simulink library "TYPEBP_MASTER_tmp"  (Simulink 8.6)
settings: Solver=ode45  StartTime=0.0  StopTime=10.0  RelTol=1e-3
undefined symbols (not defined in the file): TYPEC, TYPEC_MASTER
libraries: cdsEpicsOut x112, cdsFilt x79, cdsTP x59, cdsFiltCtrl x36, VIS_LIB x20, cdsEpicsIn x18, cdsMuxMatrix x14, STATE_BIO_MASTER x12, cdsEpicsBinIn x8, cdsFunctionCall x4, lockin x4, cdsEpicsStringIn x2
(part 2 of 13)

== system TYPEBP_MASTER_tmp/TYPEBPMASTER/TEST ==
  In1 : Inport
  In4 : Inport  Port=2
  In7 : Inport  Port=3
  In10 : Inport  Port=4
  CH1 : cdsFiltCtrl/IIR FM with control  Tag=cdsFiltCtrl  Description=|
      | cdsFiltCntrl is the standard IIR filter module (exactly the same as cdsFilt) but with added control data output 'Ctrl'. Filter module digital signal output appears on the first output, which is called 'Val'. 'Ctrl' output has a bit pattern encoding the state of filter's on/off switches (FM1 through FM10). The bit values are:
      |                                                                                                                                                                                                                                                                                                                                       
      | module 	hex	dec                                                                                                                                                                                                                                                                                                                       
      | -----------------------                                                                                                                                                                                                                                                                                                               
      | FM1	0x20                    32                                                                                                                                                                                                                                                                                                        
      | FM2	0x80                     128                                                                                                                                                                                                                                                                                                      
      | FM3	0x200                   512                                                                                                                                                                                                                                                                                                       
      | FM4	0x800                   2048                                                                                                                                                                                                                                                                                                      
      | FM5	0x2000                 8192                                                                                                                                                                                                                                                                                                       
      | FM6	0x8000                 32768                                                                                                                                                                                                                                                                                                      
      | FM7	0x20000                131072                                                                                                                                                                                                                                                                                                     
      | FM8	0x80000                 524288                                                                                                                                                                                                                                                                                                    
      | FM9	0x200000               2097152                                                                                                                                                                                                                                                                                                    
      | FM10	0x800000               8388608                                                                                                                                                                                                                                                                                                   
      |                                                                                                                                                                                                                                                                                                                                       
      | This bit data can be used to drive some other switches or it can be output using a binary I/O module.
      settings: AttributesFormatString=%<Tag>
  CH2 : cdsFiltCtrl/IIR FM with control  Tag=cdsFiltCtrl  Description=|
      | cdsFiltCntrl is the standard IIR filter module (exactly the same as cdsFilt) but with added control data output 'Ctrl'. Filter module digital signal output appears on the first output, which is called 'Val'. 'Ctrl' output has a bit pattern encoding the state of filter's on/off switches (FM1 through FM10). The bit values are:
      |                                                                                                                                                                                                                                                                                                                                       
      | module 	hex	dec                                                                                                                                                                                                                                                                                                                       
      | -----------------------                                                                                                                                                                                                                                                                                                               
      | FM1	0x20                    32                                                                                                                                                                                                                                                                                                        
      | FM2	0x80                     128                                                                                                                                                                                                                                                                                                      
      | FM3	0x200                   512                                                                                                                                                                                                                                                                                                       
      | FM4	0x800                   2048                                                                                                                                                                                                                                                                                                      
      | FM5	0x2000                 8192                                                                                                                                                                                                                                                                                                       
      | FM6	0x8000                 32768                                                                                                                                                                                                                                                                                                      
      | FM7	0x20000                131072                                                                                                                                                                                                                                                                                                     
      | FM8	0x80000                 524288                                                                                                                                                                                                                                                                                                    
      | FM9	0x200000               2097152                                                                                                                                                                                                                                                                                                    
      | FM10	0x800000               8388608                                                                                                                                                                                                                                                                                                   
      |                                                                                                                                                                                                                                                                                                                                       
      | This bit data can be used to drive some other switches or it can be output using a binary I/O module.
      settings: AttributesFormatString=%<Tag>
  CH3 : cdsFiltCtrl/IIR FM with control  Tag=cdsFiltCtrl  Description=|
      | cdsFiltCntrl is the standard IIR filter module (exactly the same as cdsFilt) but with added control data output 'Ctrl'. Filter module digital signal output appears on the first output, which is called 'Val'. 'Ctrl' output has a bit pattern encoding the state of filter's on/off switches (FM1 through FM10). The bit values are:
      |                                                                                                                                                                                                                                                                                                                                       
      | module 	hex	dec                                                                                                                                                                                                                                                                                                                       
      | -----------------------                                                                                                                                                                                                                                                                                                               
      | FM1	0x20                    32                                                                                                                                                                                                                                                                                                        
      | FM2	0x80                     128                                                                                                                                                                                                                                                                                                      
      | FM3	0x200                   512                                                                                                                                                                                                                                                                                                       
      | FM4	0x800                   2048                                                                                                                                                                                                                                                                                                      
      | FM5	0x2000                 8192                                                                                                                                                                                                                                                                                                       
      | FM6	0x8000                 32768                                                                                                                                                                                                                                                                                                      
      | FM7	0x20000                131072                                                                                                                                                                                                                                                                                                     
      | FM8	0x80000                 524288                                                                                                                                                                                                                                                                                                    
      | FM9	0x200000               2097152                                                                                                                                                                                                                                                                                                    
      | FM10	0x800000               8388608                                                                                                                                                                                                                                                                                                   
      |                                                                                                                                                                                                                                                                                                                                       
      | This bit data can be used to drive some other switches or it can be output using a binary I/O module.
      settings: AttributesFormatString=%<Tag>
  CH4 : cdsFiltCtrl/IIR FM with control  Tag=cdsFiltCtrl  Description=|
      | cdsFiltCntrl is the standard IIR filter module (exactly the same as cdsFilt) but with added control data output 'Ctrl'. Filter module digital signal output appears on the first output, which is called 'Val'. 'Ctrl' output has a bit pattern encoding the state of filter's on/off switches (FM1 through FM10). The bit values are:
      |                                                                                                                                                                                                                                                                                                                                       
      | module 	hex	dec                                                                                                                                                                                                                                                                                                                       
      | -----------------------                                                                                                                                                                                                                                                                                                               
      | FM1	0x20                    32                                                                                                                                                                                                                                                                                                        
      | FM2	0x80                     128                                                                                                                                                                                                                                                                                                      
      | FM3	0x200                   512                                                                                                                                                                                                                                                                                                       
      | FM4	0x800                   2048                                                                                                                                                                                                                                                                                                      
      | FM5	0x2000                 8192                                                                                                                                                                                                                                                                                                       
      | FM6	0x8000                 32768                                                                                                                                                                                                                                                                                                      
      | FM7	0x20000                131072                                                                                                                                                                                                                                                                                                     
      | FM8	0x80000                 524288                                                                                                                                                                                                                                                                                                    
      | FM9	0x200000               2097152                                                                                                                                                                                                                                                                                                    
      | FM10	0x800000               8388608                                                                                                                                                                                                                                                                                                   
      |                                                                                                                                                                                                                                                                                                                                       
      | This bit data can be used to drive some other switches or it can be output using a binary I/O module.
      settings: AttributesFormatString=%<Tag>
  Ground{1..6,19,22} (8 alike) : Ground
  Terminator{1..5,16..18} (8 alike) : Terminator
  wires:
  CH1/1 -> Terminator5/1
  CH3/1 -> Terminator3/1
  CH4/1 -> Terminator2/1
  In4/1 -> CH2/1
  CH2/1 -> Terminator4/1
  In1/1 -> CH1/1
  In7/1 -> CH3/1
  In10/1 -> CH4/1
  Ground22/1 -> CH1/2
  Ground19/1 -> CH1/3
  CH1/2 -> Terminator16/1
  CH2/2 -> Terminator17/1
  CH3/2 -> Terminator18/1
  Ground2/1 -> CH2/2
  Ground1/1 -> CH2/3
  Ground4/1 -> CH3/2
  Ground3/1 -> CH3/3
  Ground6/1 -> CH4/2
  Ground5/1 -> CH4/3
  CH4/2 -> Terminator1/1

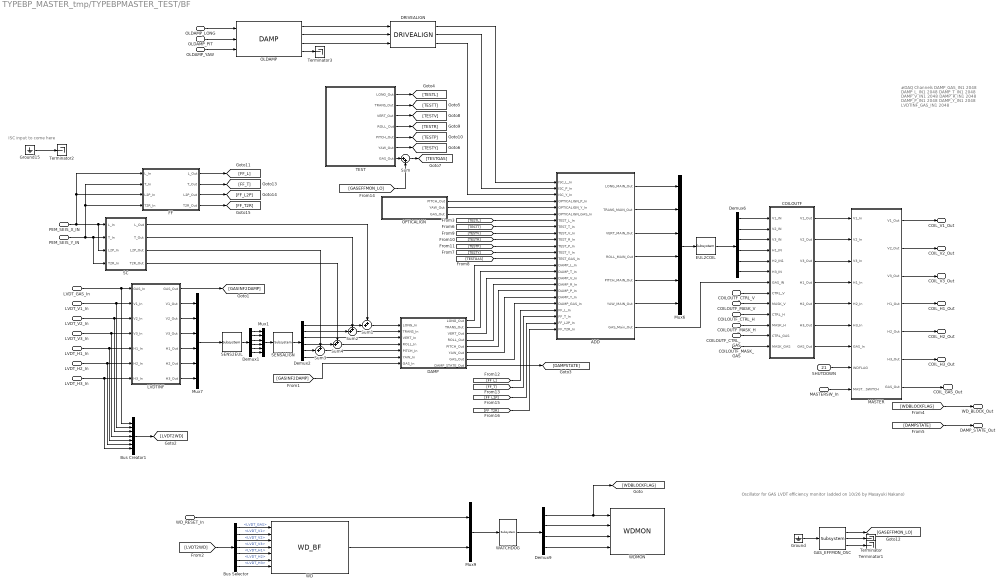
== system TYPEBP_MASTER_tmp/TYPEBPMASTER_TEST/BF ==
  note: #DAQ Channels
      | DAMP_GAS_IN1 2048
      | DAMP_L_IN1 2048
      | DAMP_T_IN1 2048
      | DAMP_V_IN1 2048
      | DAMP_R_IN1 2048
      | DAMP_P_IN1 2048
      | DAMP_Y_IN1 2048
      | LVDTINF_GAS_IN1 2048
  note: ISC input to come here
  note: Oscillator for GAS LVDT efficiency monitor (added on 10/26 by Masayuki Nakano)
  LVDT_GAS_In : Inport
  LVDT_V1_In : Inport  Port=2
  LVDT_V2_In : Inport  Port=3
  LVDT_V3_In : Inport  Port=4
  LVDT_H1_In : Inport  Port=5
  LVDT_H2_In : Inport  Port=6
  LVDT_H3_In : Inport  Port=7
  COILOUTF_CTRL_V : Inport  Port=8
  COILOUTF_MASK_V : Inport  Port=9
  COILOUTF_CTRL_H : Inport  Port=10
  COILOUTF_MASK_H : Inport  Port=11
  COILOUTF_CTRL_GAS : Inport  Port=12
  COILOUTF_MASK_GAS : Inport  Port=13
  MASTERSW_In : Inport  Port=14
  WD_RESET_In : Inport  Port=15
  OLDAMP_LONG : Inport  Port=16
  OLDAMP_PIT : Inport  Port=17
  OLDAMP_YAW : Inport  Port=18
  PEM_SEIS_X_IN : Inport  Port=19
  PEM_SEIS_Y_IN : Inport  Port=20
  SHUTDOWN : Inport  Port=21
  ADD : Subsystem
  Bus Creator1 : BusCreator  Inputs='LVDT_GAS','LVDT_V1','LVDT_V2','LVDT_V3','LVDT_H1','LVDT_H2','LVDT_H3'
  Bus Selector : BusSelector  OutputSignals=LVDT_GAS,LVDT_V1,LVDT_V2,LVDT_V3,LVDT_H1,LVDT_H2,LVDT_H3
  COILOUTF : Subsystem
  DAMP : Subsystem
  DRIVEALIGN : CRYP_IM_MASTER/CRYP_IM_MASTER/DRIVEALIGN
  Demux1 : Demux  Outputs=6
  Demux2 : Demux  Outputs=6
  Demux6 : Demux  Outputs=6
  Demux9 : Demux
  EUL2COIL : cdsMuxMatrix/Subsystem  Tag=cdsMuxMatrix  Description=|
      | ADL=SUS_INMATRIX.adl
      | SCRIPT=generate_KisselButton.py 4 5 #CHANNEL# > #TARGET_DIR#/#FULL_PART_NAME#_KB.adl
      settings: AttributesFormatString=%<Tag>
  FF : Subsystem  AncestorBlock=TYPEBP_MASTER/TYPEBPMASTER_TEST/SF/FF
  GAS_EFFMON_OSC : cdsOsc/Subsystem  Tag=cdsOsc  Description=Oscillator
      settings: AttributesFormatString=%<Tag>
  Ground : Ground
  Ground15 : Ground
  LVDTINF : Subsystem
  MASTER : Subsystem
  Mux1 : Mux  Inputs=6
  Mux6 : Mux  Inputs=6
  Mux7 : Mux  Inputs=6
  Mux9 : Mux  Inputs=2
  OLDAMP : VIS_LIB/DAMP
  OPTICALIGN : Subsystem
  SC : Subsystem
  SENS2EUL : cdsMuxMatrix/Subsystem  Tag=cdsMuxMatrix  Description=Any size matrix. Inputs and outputs must be connected using Mux and Demux parts.
      settings: AttributesFormatString=%<Tag>
  SENSALIGN : cdsMuxMatrix/Subsystem  Tag=cdsMuxMatrix  Description=Any size matrix. Inputs and outputs must be connected using Mux and Demux parts.
      settings: AttributesFormatString=%<Tag>
  Sum : Sum  Inputs=|++
  Sum{1..4} (4 alike) : Sum  Inputs=++|
  TEST : Subsystem
  Terminator{,1..3} (4 alike) : Terminator
  WATCHDOG : cdsFunctionCall/Subsystem  Tag=cdsFunctionCall  Description=inline OSEMWATCHDOG /opt/rtcds/userapps/release/vis/common/src/WATCHDOG.c
      settings: AttributesFormatString=%<Tag>\n%<Description>
  WD : VIS_LIB/WD_BF
  WDMON : SIXOSEM_F_STAGE_MASTER/SIXOSEM_F_STAGE_MASTER/WDMON
  COIL_GAS_Out : Outport
  COIL_V1_Out : Outport  Port=2
  COIL_V2_Out : Outport  Port=3
  COIL_V3_Out : Outport  Port=4
  COIL_H1_Out : Outport  Port=5
  COIL_H2_Out : Outport  Port=6
  COIL_H3_Out : Outport  Port=7
  WD_BLOCK_Out : Outport  Port=8
  DAMP_STATE_Out : Outport  Port=9
  wires:
  SC/4(T2R_Out) -> Sum4/1
  Sum4/1 -> DAMP/4(ROLL_In)
  SC/3(L2P_Out) -> Sum3/1
  Sum3/1 -> DAMP/5(PITCH_In)
  [FF_T2R] -> ADD/24(FF_T2R_In)
  [FF_L2P] -> ADD/23(FF_L2P_In)
  FF/4(T2R_Out) -> [FF_T2R]
  FF/3(L2P_Out) -> [FF_L2P]
  [FF_T] -> ADD/22(FF_T_In)
  [FF_L] -> ADD/21(FF_L_In)
  FF/2(T_Out) -> [FF_T]
  FF/1(L_Out) -> [FF_L]
  PEM_SEIS_X_IN/1 -> SC/1(L_In), SC/3(L2P_In), FF/3(L2P_In), FF/1(L_In)
  Sum2/1 -> DAMP/2(TRANS_In)
  Sum1/1 -> DAMP/1(LONG_In)
  SC/2(T_Out) -> Sum2/1
  PEM_SEIS_Y_IN/1 -> FF/2(T_In), FF/4(T2R_In), SC/2(T_In), SC/4(T2R_In)
  SC/1(L_Out) -> Sum1/1
  DRIVEALIGN/1 -> ADD/1(ISC_L_In)
  DRIVEALIGN/2 -> ADD/2(ISC_P_In)
  DRIVEALIGN/3 -> ADD/3(ISC_Y_In)
  OLDAMP/3 -> DRIVEALIGN/3
  OLDAMP/2 -> DRIVEALIGN/2
  OLDAMP/1 -> DRIVEALIGN/1
  Ground15/1 -> Terminator2/1
  OLDAMP_LONG/1 -> OLDAMP/1
  OLDAMP_PIT/1 -> OLDAMP/2
  OLDAMP_YAW/1 -> OLDAMP/3
  OLDAMP/4 -> Terminator3/1
  GAS_EFFMON_OSC/3 -> Terminator1/1
  GAS_EFFMON_OSC/2 -> Terminator/1
  Ground/1 -> GAS_EFFMON_OSC/1
  [GASEFFMON_LO] -> Sum/2
  Sum/1 -> [TESTGAS]
  TEST/7(GAS_Out) -> Sum/1
  GAS_EFFMON_OSC/1 -> [GASEFFMON_LO]
  [GASINF2DAMP] -> DAMP/7(GAS_In)
  COILOUTF_MASK_GAS/1 -> COILOUTF/13(MASK_GAS)
  COILOUTF_CTRL_GAS/1 -> COILOUTF/12(CTRL_GAS)
  COILOUTF_MASK_H/1 -> COILOUTF/11(MASK_H)
  COILOUTF_CTRL_H/1 -> COILOUTF/10(CTRL_H)
  LVDTINF/7(H3_Out) -> Mux7/6
  LVDTINF/6(H2_Out) -> Mux7/5
  LVDTINF/5(H1_Out) -> Mux7/4
  Bus Selector/7 -> WD/7  "<LVDT_H3>"
  Bus Selector/6 -> WD/6  "<LVDT_H2>"
  Bus Selector/5 -> WD/5  "<LVDT_H1>"
  Bus Selector/4 -> WD/4  "<LVDT_V3>"
  Bus Selector/3 -> WD/3  "<LVDT_V2>"
  Bus Selector/2 -> WD/2  "<LVDT_V1>"
  [DAMPSTATE] -> DAMP_STATE_Out/1
  [WDBLOCKFLAG] -> WD_BLOCK_Out/1
  MASTER/7(GAS_Out) -> COIL_GAS_Out/1
  MASTER/6(H3_Out) -> COIL_H3_Out/1
  MASTER/5(H2_Out) -> COIL_H2_Out/1
  MASTERSW_In/1 -> MASTER/9(MASTERSWITCH)
  SHUTDOWN/1 -> MASTER/8(WDFLAG)
  COILOUTF/4(H1_Out) -> MASTER/4(H1_In)
  COILOUTF/3(V3_Out) -> MASTER/3(V3_In)
  COILOUTF/2(V2_Out) -> MASTER/2(V2_In)
  COILOUTF/1(V1_Out) -> MASTER/1(V1_In)
  COILOUTF/7(GAS_Out) -> MASTER/7(GAS_In)
  COILOUTF/6(H3_Out) -> MASTER/6(H3_In)
  COILOUTF/5(H2_Out) -> MASTER/5(H2_In)
  Demux6/6 -> COILOUTF/6(H3_IN)
  Demux6/5 -> COILOUTF/5(H2_IN1)
  Demux6/4 -> COILOUTF/4(H1_IN)
  Demux6/3 -> COILOUTF/3(V3_IN)
  Demux6/2 -> COILOUTF/2(V2_IN)
  Demux6/1 -> COILOUTF/1(V1_IN)
  OPTICALIGN/3(GAS_Out) -> ADD/6(OPTICALIGN_GAS_In)
  OPTICALIGN/2(YAW_Out) -> ADD/5(OPTICALIGN_Y_In)
  OPTICALIGN/1(PITCH_Out) -> ADD/4(OPTICALIGN_P_In)
  ADD/1(LONG_MAIN_Out) -> Mux6/1
  ADD/2(TRANS_MAIN_Out) -> Mux6/2
  ADD/3(VERT_MAIN_Out) -> Mux6/3
  ADD/4(ROLL_MAIN_Out) -> Mux6/4
  ADD/5(PITCH_MAIN_Out) -> Mux6/5
  ADD/6(YAW_MAIN_Out) -> Mux6/6
  ADD/7(GAS_Main_Out) -> COILOUTF/7(GAS_IN)
  DAMP/1(LONG_Out) -> ADD/14(DAMP_L_In)
  DAMP/2(TRANS_Out) -> ADD/15(DAMP_T_In)
  DAMP/3(VERT_Out) -> ADD/16(DAMP_V_In)
  DAMP/4(ROLL_Out) -> ADD/17(DAMP_R_In)
  DAMP/5(PITCH_Out) -> ADD/18(DAMP_P_In)
  DAMP/6(YAW_Out) -> ADD/19(DAMP_Y_In)
  DAMP/7(GAS_Out) -> ADD/20(DAMP_GAS_In)
  [TESTP] -> ADD/11(TEST_P_In)
  [TESTR] -> ADD/10(TEST_R_In)
  [TESTV] -> ADD/9(TEST_V_In)
  TEST/5(PITCH_Out) -> [TESTP]
  TEST/4(ROLL_Out) -> [TESTR]
  TEST/3(VERT_Out) -> [TESTV]
  DAMP/8(DAMP_STATE_Out) -> [DAMPSTATE]
  LVDTINF/4(V3_Out) -> Mux7/3
  LVDTINF/3(V2_Out) -> Mux7/2
  LVDTINF/2(V1_Out) -> Mux7/1
  SENSALIGN/1 -> Demux2/1
  Mux1/1 -> SENSALIGN/1
  Demux1/6 -> Mux1/6
  Demux1/5 -> Mux1/5
  Demux1/4 -> Mux1/4
  Demux1/3 -> Mux1/3
  Demux1/2 -> Mux1/2
  Demux1/1 -> Mux1/1
  SENS2EUL/1 -> Demux1/1
  Demux2/1 -> Sum1/2
  Demux2/2 -> Sum2/2
  Demux2/3 -> DAMP/3(VERT_In)
  Demux2/4 -> Sum4/2
  Demux2/5 -> Sum3/2
  Demux2/6 -> DAMP/6(YAW_In)
  Bus Selector/1 -> WD/1  "<LVDT_GAS>"
  MASTER/4(H1_Out) -> COIL_H1_Out/1
  [TESTGAS] -> ADD/13(TEST_GAS_In)
  [TESTY] -> ADD/12(TEST_Y_In)
  [TESTT] -> ADD/8(TEST_T_In)
  [TESTL] -> ADD/7(TEST_L_In)
  TEST/6(YAW_Out) -> [TESTY]
  TEST/2(TRANS_Out) -> [TESTT]
  TEST/1(LONG_Out) -> [TESTL]
  LVDTINF/1(GAS_Out) -> [GASINF2DAMP]
  LVDT_GAS_In/1 -> LVDTINF/1(GAS_In), Bus Creator1/1
  COILOUTF_MASK_V/1 -> COILOUTF/9(MASK_V)
  COILOUTF_CTRL_V/1 -> COILOUTF/8(CTRL_V)
  Bus Creator1/1 -> [LVDT2WD]
  LVDT_H3_In/1 -> Bus Creator1/7, LVDTINF/7(H3_In)
  LVDT_H2_In/1 -> Bus Creator1/6, LVDTINF/6(H2_In)
  LVDT_H1_In/1 -> Bus Creator1/5, LVDTINF/5(H1_In)
  LVDT_V3_In/1 -> LVDTINF/4(V3_In), Bus Creator1/4
  LVDT_V2_In/1 -> LVDTINF/3(V2_In), Bus Creator1/3
  LVDT_V1_In/1 -> LVDTINF/2(V1_In), Bus Creator1/2
  WATCHDOG/1 -> Demux9/1
  Mux9/1 -> WATCHDOG/1
  Demux9/4 -> WDMON/4
  Demux9/3 -> WDMON/3
  Demux9/2 -> WDMON/2
  Demux9/1 -> WDMON/1, [WDBLOCKFLAG]
  [LVDT2WD] -> Bus Selector/1
  WD/1 -> Mux9/2
  WD_RESET_In/1 -> Mux9/1
  MASTER/3(V3_Out) -> COIL_V3_Out/1
  MASTER/2(V2_Out) -> COIL_V2_Out/1
  MASTER/1(V1_Out) -> COIL_V1_Out/1
  EUL2COIL/1 -> Demux6/1
  Mux6/1 -> EUL2COIL/1
  Mux7/1 -> SENS2EUL/1

== system TYPEBP_MASTER_tmp/TYPEBPMASTER_TEST/BIO ==
  note: 12 Bit Word
  note: 12 Bit Word
  note: 12 Bit Word
  note: 12 Bit Word
  note: 12 Bit Word
  TM_ISC_CTRL : Inport
  TM_MON_In : Inport  Port=2
  IM1_CTRL : Inport  Port=3
  IM1_MON_In : Inport  Port=4
  IM2_ISC_CTRL : Inport  Port=5
  IM2_MON_In : Inport  Port=6
  GAS_ISC_CTRL : Inport  Port=7
  GAS_MON_In : Inport  Port=8
  BFV_ISC_CTRL : Inport  Port=9
  BFV_MON_In : Inport  Port=10
  BFH_ISC_CTRL : Inport  Port=11
  BFH_MON_In : Inport  Port=12
  BFH : STATE_BIO_MASTER/UIM_BIO_MASTER
  BFV : STATE_BIO_MASTER/UIM_BIO_MASTER
  GAS : STATE_BIO_MASTER/UIM_BIO_MASTER
  IM1 : STATE_BIO_MASTER/UIM_BIO_MASTER
  IM2 : STATE_BIO_MASTER/UIM_BIO_MASTER
  TM : STATE_BIO_MASTER/UIM_BIO_MASTER
  TM_BO_CTRL_Out : Outport
  TM_MASK_Out : Outport  Port=2
  TM_CTRL_Out : Outport  Port=3
  IM1_BO_CTRL_Out : Outport  Port=4
  IM1_MASK_Out : Outport  Port=5
  IM1_CTRL_Out : Outport  Port=6
  IM2_BO_CTRL_Out : Outport  Port=7
  IM2_MASK_Out : Outport  Port=8
  IM2_CTRL_Out : Outport  Port=9
  GAS_BO_CTRL_Out : Outport  Port=10
  GAS_MASK_Out : Outport  Port=11
  GAS_CTRL_Out : Outport  Port=12
  BFV_BO_CTRL_Out : Outport  Port=13
  BFV_MASK_Out : Outport  Port=14
  BFV_CTRL_Out : Outport  Port=15
  BFH_BO_CTRL_Out : Outport  Port=16
  BFH_MASK_Out : Outport  Port=17
  BFH_CTRL_Out : Outport  Port=18
  wires:
  BFH_MON_In/1 -> BFH/2
  BFH_ISC_CTRL/1 -> BFH/1
  BFH/1 -> BFH_MASK_Out/1
  BFH/2 -> BFH_CTRL_Out/1
  BFH/3 -> BFH_BO_CTRL_Out/1
  TM_MON_In/1 -> TM/2
  TM_ISC_CTRL/1 -> TM/1
  IM1_CTRL/1 -> IM1/1
  IM1_MON_In/1 -> IM1/2
  IM2_MON_In/1 -> IM2/2
  IM2_ISC_CTRL/1 -> IM2/1
  GAS_MON_In/1 -> GAS/2
  GAS_ISC_CTRL/1 -> GAS/1
  BFV_MON_In/1 -> BFV/2
  BFV_ISC_CTRL/1 -> BFV/1
  TM/1 -> TM_MASK_Out/1
  TM/2 -> TM_CTRL_Out/1
  TM/3 -> TM_BO_CTRL_Out/1
  IM1/1 -> IM1_MASK_Out/1
  IM1/2 -> IM1_CTRL_Out/1
  IM1/3 -> IM1_BO_CTRL_Out/1
  IM2/1 -> IM2_MASK_Out/1
  IM2/2 -> IM2_CTRL_Out/1
  IM2/3 -> IM2_BO_CTRL_Out/1
  GAS/1 -> GAS_MASK_Out/1
  GAS/2 -> GAS_CTRL_Out/1
  GAS/3 -> GAS_BO_CTRL_Out/1
  BFV/1 -> BFV_MASK_Out/1
  BFV/2 -> BFV_CTRL_Out/1
  BFV/3 -> BFV_BO_CTRL_Out/1

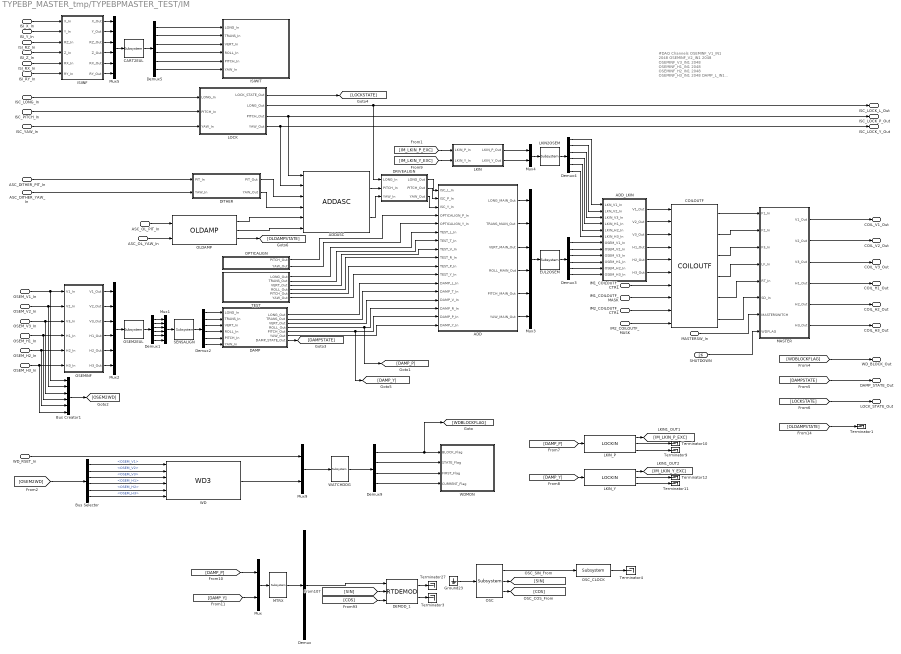
== system TYPEBP_MASTER_tmp/TYPEBPMASTER_TEST/IM ==
  note: #DAQ Channels
      | OSEMINF_V1_IN1 2048
      | OSEMINF_V2_IN1 2048
      | OSEMINF_V3_IN1 2048
      | OSEMINF_H1_IN1 2048
      | OSEMINF_H2_IN1 2048
      | OSEMINF_H3_IN1 2048
      | DAMP_L_IN1 2048
      | DAMP_T_IN1 2048
      | DAMP_V_IN1 2048
      | DAMP_R_IN1 2048
      | DAMP_P_IN1 2048
      | DAMP_Y_IN1 2048
  ISI_X_In : Inport
  ISI_Y_In : Inport  Port=2
  ISI_RZ_In : Inport  Port=3
  ISI_Z_In : Inport  Port=4
  ISI_RX_In : Inport  Port=5
  ISI_RY_In : Inport  Port=6
  OSEM_V1_In : Inport  Port=7
  OSEM_V2_In : Inport  Port=8
  OSEM_V3_In : Inport  Port=9
  OSEM_H1_In : Inport  Port=10
  OSEM_H2_In : Inport  Port=11
  OSEM_H3_In : Inport  Port=12
  ISC_LONG_In : Inport  Port=13
  ISC_PITCH_In : Inport  Port=14
  ISC_YAW_In : Inport  Port=15
  ASC_DITHER_PIT_In : Inport  Port=16
  ASC_DITHER_YAW_In : Inport  Port=17
  IM1_COILOUTF_CTRL : Inport  Port=18
  IM1_COILOUTF_MASK : Inport  Port=19
  IM2_COILOUTF_CTRL : Inport  Port=20
  IM2_COILOUTF_MASK : Inport  Port=21
  MASTERSW_In : Inport  Port=22
  WD_RSET_In : Inport  Port=23
  ASC_OL_PIT_In : Inport  Port=24
  ASC_OL_YAW_In : Inport  Port=25
  SHUTDOWN : Inport  Port=26
  ADD : Subsystem
  ADDASC : VIS_LIB/ADDASC
  ADD_LKIN : Subsystem
  Bus Creator1 : BusCreator  Inputs='OSEM_V1','OSEM_V2','OSEM_V3','OSEM_H1','OSEM_H2','OSEM_H3'
  Bus Selector : BusSelector  OutputSignals=OSEM_V1,OSEM_V2,OSEM_V3,OSEM_H1,OSEM_H2,OSEM_H3
  CART2EUL : cdsMuxMatrix/Subsystem  Tag=cdsMuxMatrix  Description=Any size matrix. Inputs and outputs must be connected using Mux and Demux parts.
      settings: AttributesFormatString=%<Tag>
  COILOUTF : SIXOSEM_F_COILOUTF_MASTER/COILOUTF
  DAMP : Subsystem
  DEMOD_1 : rtdemod/RTDEMOD  Tag=top_names
  DITHER : Subsystem
  DRIVEALIGN : Subsystem
  Demux : Demux  Outputs=1
  Demux{1..5} (5 alike) : Demux  Outputs=6
  Demux9 : Demux
  EUL2OSEM : cdsMuxMatrix/Subsystem  Tag=cdsMuxMatrix  Description=Any size matrix. Inputs and outputs must be connected using Mux and Demux parts.
      settings: AttributesFormatString=%<Tag>
  Ground23 : Ground
  ISIINF : Subsystem
  ISIWIT : Subsystem
  LKIN : Subsystem
  LKIN2OSEM : cdsMuxMatrix/Subsystem  Tag=cdsMuxMatrix  Description=Any size matrix. Inputs and outputs must be connected using Mux and Demux parts.
      settings: AttributesFormatString=%<Tag>
  LKIN_P : lockin/LOCKIN  Description=ADL=LOCKIN.adl
      settings: AttributesFormatString=%<Tag>
  LKIN_Y : lockin/LOCKIN  Description=ADL=LOCKIN.adl
      settings: AttributesFormatString=%<Tag>
  LOCK : Subsystem
  MASTER : Subsystem
  MTRX : cdsMuxMatrix/Subsystem  Tag=cdsMuxMatrix  Description=Any size matrix. Inputs and outputs must be connected using Mux and Demux parts.
      settings: AttributesFormatString=%<Tag>
  Mux : Mux  Inputs=2
  Mux{1..3,5} (4 alike) : Mux  Inputs=6
  Mux4 : Mux  Inputs=2
  Mux9 : Mux  Inputs=2
  OLDAMP : VIS_LIB/OLDAMP
  OPTICALIGN : Subsystem
  OSC : cdsOsc/Subsystem  Tag=cdsOsc  Description=Oscillator
      settings: AttributesFormatString=%<Tag>
  OSC_CLOCK : cdsEpicsOut/Subsystem  Tag=cdsEpicsOutput  Description=|
      | Purpose:                                          
      | Output a FE signal to an EPICS channel.           
      |                                                   
      | Operation:                                        
      | Takes input value and passes it to EPICS record.  
      |                                                   
      | Usage:                                            
      | Name the part with the desired EPICS rrecord name.
      settings: AttributesFormatString=%<Tag>
  OSEM2EUL : cdsMuxMatrix/Subsystem  Tag=cdsMuxMatrix  Description=Any size matrix. Inputs and outputs must be connected using Mux and Demux parts.
      settings: AttributesFormatString=%<Tag>
  OSEMINF : Subsystem
  SENSALIGN : cdsMuxMatrix/Subsystem  Tag=cdsMuxMatrix  Description=Any size matrix. Inputs and outputs must be connected using Mux and Demux parts.
      settings: AttributesFormatString=%<Tag>
  TEST : Subsystem
  Terminator{1,3..4,9..12,27} (8 alike) : Terminator
  WATCHDOG : cdsFunctionCall/Subsystem  Tag=cdsFunctionCall  Description=inline OSEMWATCHDOG /opt/rtcds/userapps/release/vis/common/src/WATCHDOG.c
      settings: AttributesFormatString=%<Tag>\n%<Description>
  WD : VIS_LIB/WD3
  WDMON : Subsystem
  ISC_LOCK_L_Out : Outport
  ISC_LOCK_P_Out : Outport  Port=2
  ISC_LOCK_Y_Out : Outport  Port=3
  COIL_V1_Out : Outport  Port=4
  COIL_V2_Out : Outport  Port=5
  COIL_V3_Out : Outport  Port=6
  COIL_H1_Out : Outport  Port=7
  COIL_H2_Out : Outport  Port=8
  COIL_H3_Out : Outport  Port=9
  WD_BLOCK_Out : Outport  Port=10
  DAMP_STATE_Out : Outport  Port=11
  LOCK_STATE_Out : Outport  Port=12
  wires:
  IM2_COILOUTF_MASK/1 -> COILOUTF/10
  IM2_COILOUTF_CTRL/1 -> COILOUTF/9
  [OLDAMPSTATE] -> Terminator1/1
  ASC_OL_PIT_In/1 -> OLDAMP/1
  ASC_OL_YAW_In/1 -> OLDAMP/2
  OLDAMP/1 -> ADDASC/5
  OLDAMP/2 -> ADDASC/6
  OLDAMP/3 -> [OLDAMPSTATE]
  Mux/1 -> MTRX/1
  MTRX/1 -> Demux/1
  Demux/1 -> DEMOD_1/1
  [SIN] -> DEMOD_1/2
  [COS] -> DEMOD_1/3
  DEMOD_1/1 -> Terminator27/1
  DEMOD_1/2 -> Terminator3/1
  Ground23/1 -> OSC/1
  OSC/1 -> OSC_CLOCK/1
  OSC_CLOCK/1 -> Terminator4/1
  OSC/2 -> [SIN]
  OSC/3 -> [COS]
  [DAMP_P] -> Mux/1
  [DAMP_Y] -> Mux/2
  [DAMP_Y] -> LKIN_Y/1
  [DAMP_P] -> LKIN_P/1
  [IM_LKIN_Y_EXC] -> LKIN/2(LKIN_Y_In)
  [IM_LKIN_P_EXC] -> LKIN/1(LKIN_P_In)
  LKIN_Y/3 -> Terminator11/1
  LKIN_Y/2 -> Terminator12/1
  LKIN_Y/1 -> [IM_LKIN_Y_EXC]
  LKIN_P/1 -> [IM_LKIN_P_EXC]
  LKIN_P/3 -> Terminator9/1
  LKIN_P/2 -> Terminator10/1
  DAMP/1(LONG_Out) -> ADD/12(DAMP_L_In)
  DAMP/2(TRANS_Out) -> ADD/13(DAMP_T_In)
  DAMP/3(VERT_Out) -> ADD/14(DAMP_V_In)
  DAMP/4(ROLL_Out) -> ADD/15(DAMP_R_In), [DAMP_P]
  DAMP/5(PITCH_Out) -> ADD/16(DAMP_P_In), [DAMP_Y]
  DAMP/6(YAW_Out) -> ADD/17(DAMP_Y_In)
  TEST/1(LONG_Out) -> ADD/6(TEST_L_In)
  TEST/2(TRANS_Out) -> ADD/7(TEST_T_In)
  TEST/3(VERT_Out) -> ADD/8(TEST_V_In)
  TEST/4(ROLL_Out) -> ADD/9(TEST_R_In)
  TEST/5(PITCH_Out) -> ADD/10(TEST_P_In)
  TEST/6(YAW_Out) -> ADD/11(TEST_Y_In)
  OPTICALIGN/1(PITCH_Out) -> ADD/4(OPTICALIGN_P_In)
  OPTICALIGN/2(YAW_Out) -> ADD/5(OPTICALIGN_Y_In)
  DITHER/1(PIT_Out) -> ADDASC/3
  DITHER/2(YAW_Out) -> ADDASC/4
  ASC_DITHER_PIT_In/1 -> DITHER/1(PIT_In)
  ASC_DITHER_YAW_In/1 -> DITHER/2(YAW_In)
  ADDASC/2 -> DRIVEALIGN/3(YAW_In)
  ADDASC/1 -> DRIVEALIGN/2(PITCH_In)
  DRIVEALIGN/1(LONG_Out) -> ADD/1(ISC_L_In)
  DRIVEALIGN/2(PITCH_Out) -> ADD/2(ISC_P_In)
  DRIVEALIGN/3(YAW_Out) -> ADD/3(ISC_Y_In)
  LOCK/4(YAW_Out) -> ISC_LOCK_Y_Out/1, ADDASC/2
  LOCK/3(PITCH_Out) -> ISC_LOCK_P_Out/1, ADDASC/1
  LOCK/2(LONG_Out) -> ISC_LOCK_L_Out/1, DRIVEALIGN/1(LONG_In)
  WD_RSET_In/1 -> Mux9/1
  WD/1 -> Mux9/2
  LKIN/2(LKIN_Y_Out) -> Mux4/2
  IM1_COILOUTF_CTRL/1 -> COILOUTF/7
  IM1_COILOUTF_MASK/1 -> COILOUTF/8
  MASTERSW_In/1 -> MASTER/7(MASTERSWITCH)
  Demux3/6 -> ADD_LKIN/12(OSEM_H3_In)
  Demux3/5 -> ADD_LKIN/11(OSEM_H2_In)
  Demux3/4 -> ADD_LKIN/10(OSEM_H1_In)
  Demux3/3 -> ADD_LKIN/9(OSEM_V3_In)
  Demux3/2 -> ADD_LKIN/8(OSEM_V2_In)
  Demux3/1 -> ADD_LKIN/7(OSEM_V1_In)
  Demux4/6 -> ADD_LKIN/6(LKIN_H3_In)
  Demux4/5 -> ADD_LKIN/5(LKIN_H2_In)
  Demux4/4 -> ADD_LKIN/4(LKIN_H1_In)
  Demux4/3 -> ADD_LKIN/3(LKIN_V3_In)
  Demux4/2 -> ADD_LKIN/2(LKN_V2_In)
  Demux4/1 -> ADD_LKIN/1(LKN_V1_In)
  ADD_LKIN/6(H3_Out) -> COILOUTF/6
  ADD_LKIN/5(H2_Out) -> COILOUTF/5
  ADD_LKIN/4(H1_Out) -> COILOUTF/4
  ADD_LKIN/3(V3_Out) -> COILOUTF/3
  ADD_LKIN/2(V2_Out) -> COILOUTF/2
  ADD_LKIN/1(V1_Out) -> COILOUTF/1
  Mux4/1 -> LKIN2OSEM/1
  LKIN2OSEM/1 -> Demux4/1
  LKIN/1(LKIN_P_Out) -> Mux4/1
  [LOCKSTATE] -> LOCK_STATE_Out/1
  LOCK/1(LOCK_STATE_Out) -> [LOCKSTATE]
  ADD/6(YAW_MAIN_Out) -> Mux3/6
  ADD/5(PITCH_MAIN_Out) -> Mux3/5
  ADD/4(ROLL_MAIN_Out) -> Mux3/4
  ADD/3(VERT_MAIN_Out) -> Mux3/3
  ADD/2(TRANS_MAIN_Out) -> Mux3/2
  ADD/1(LONG_MAIN_Out) -> Mux3/1
  [DAMPSTATE] -> DAMP_STATE_Out/1
  DAMP/7(DAMP_STATE_Out) -> [DAMPSTATE]
  [WDBLOCKFLAG] -> WD_BLOCK_Out/1
  Demux2/6 -> DAMP/6(YAW_In)
  Demux2/5 -> DAMP/5(PITCH_In)
  Demux2/4 -> DAMP/4(ROLL_In)
  Demux2/3 -> DAMP/3(VERT_In)
  Demux2/2 -> DAMP/2(TRANS_In)
  Demux2/1 -> DAMP/1(LONG_In)
  SHUTDOWN/1 -> MASTER/8(WDFLAG)
  Demux5/6 -> ISIWIT/6(YAW_In)
  Demux5/5 -> ISIWIT/5(PITCH_In)
  Demux5/4 -> ISIWIT/4(ROLL_In)
  Demux5/3 -> ISIWIT/3(VERT_In)
  Demux5/2 -> ISIWIT/2(TRANS_In)
  Demux5/1 -> ISIWIT/1(LONG_In)
  CART2EUL/1 -> Demux5/1
  Mux5/1 -> CART2EUL/1
  ISIINF/6(RY_Out) -> Mux5/6
  ISIINF/5(RX_Out) -> Mux5/5
  ISIINF/4(Z_Out) -> Mux5/4
  ISIINF/3(RZ_Out) -> Mux5/3
  ISIINF/2(Y_Out) -> Mux5/2
  ISIINF/1(X_Out) -> Mux5/1
  ISI_RY_In/1 -> ISIINF/6(RY_In)
  ISI_RX_In/1 -> ISIINF/5(RX_In)
  ISI_Z_In/1 -> ISIINF/4(Z_In)
  ISI_RZ_In/1 -> ISIINF/3(RZ_In)
  ISI_Y_In/1 -> ISIINF/2(Y_In)
  ISI_X_In/1 -> ISIINF/1(X_In)
  OSEMINF/6(H3_Out) -> Mux2/6
  OSEMINF/5(H2_Out) -> Mux2/5
  OSEMINF/4(H1_Out) -> Mux2/4
  OSEMINF/3(V3_Out) -> Mux2/3
  OSEMINF/2(V2_Out) -> Mux2/2
  OSEMINF/1(V1_Out) -> Mux2/1
  OSEM_V1_In/1 -> OSEMINF/1(V1_In), Bus Creator1/1
  OSEM_V2_In/1 -> OSEMINF/2(V2_In), Bus Creator1/2
  OSEM_V3_In/1 -> OSEMINF/3(V3_In), Bus Creator1/3
  OSEM_H1_In/1 -> OSEMINF/4(H1_In), Bus Creator1/4
  OSEM_H2_In/1 -> OSEMINF/5(H2_In), Bus Creator1/5
  OSEM_H3_In/1 -> OSEMINF/6(H3_In), Bus Creator1/6
  Mux2/1 -> OSEM2EUL/1
  ISC_LONG_In/1 -> LOCK/1(LONG_In)
  ISC_PITCH_In/1 -> LOCK/2(PITCH_In)
  ISC_YAW_In/1 -> LOCK/3(YAW_In)
  Bus Creator1/1 -> [OSEM2WD]
  [OSEM2WD] -> Bus Selector/1
  Bus Selector/1 -> WD/1  "<OSEM_V1>"
  Bus Selector/2 -> WD/2  "<OSEM_V2>"
  Bus Selector/3 -> WD/3  "<OSEM_V3>"
  Bus Selector/4 -> WD/4  "<OSEM_H1>"
  Bus Selector/5 -> WD/5  "<OSEM_H2>"
  Bus Selector/6 -> WD/6  "<OSEM_H3>"
  OSEM2EUL/1 -> Demux1/1
  Demux1/1 -> Mux1/1
  Demux1/2 -> Mux1/2
  Demux1/3 -> Mux1/3
  Demux1/4 -> Mux1/4
  Demux1/5 -> Mux1/5
  Demux1/6 -> Mux1/6
  Mux1/1 -> SENSALIGN/1
  SENSALIGN/1 -> Demux2/1
  MASTER/1(V1_Out) -> COIL_V1_Out/1
  MASTER/2(V2_Out) -> COIL_V2_Out/1
  MASTER/3(V3_Out) -> COIL_V3_Out/1
  MASTER/4(H1_Out) -> COIL_H1_Out/1
  MASTER/5(H2_Out) -> COIL_H2_Out/1
  MASTER/6(H3_Out) -> COIL_H3_Out/1
  Mux3/1 -> EUL2OSEM/1
  EUL2OSEM/1 -> Demux3/1
  Demux9/1 -> [WDBLOCKFLAG], WDMON/1(BLOCK_Flag)
  Demux9/2 -> WDMON/2(STATE_Flag)
  Demux9/3 -> WDMON/3(FIRST_Flag)
  Demux9/4 -> WDMON/4(CURRENT_Flag)
  COILOUTF/1 -> MASTER/1(F1_In)
  COILOUTF/2 -> MASTER/2(F2_In)
  COILOUTF/3 -> MASTER/3(F3_In)
  COILOUTF/4 -> MASTER/4(LF_In)
  COILOUTF/5 -> MASTER/5(RT_In)
  COILOUTF/6 -> MASTER/6(SD_In)
  Mux9/1 -> WATCHDOG/1
  WATCHDOG/1 -> Demux9/1

== system TYPEBP_MASTER_tmp/TYPEBPMASTER_TEST/SF ==
  note: #DAQ Channels
      | LVDTINF_GAS_IN1 2048
      | DAMP_GAS_IN1 2048
  LVDT_GAS_IN : Inport
  COILOUT_CTRL : Inport  Port=2
  COILOUTF_MASK : Inport  Port=3
  MASTERSW_IN : Inport  Port=4
  WDRESET_IN : Inport  Port=5
  PEM_SEIS_Z_IN : Inport  Port=6
  SHUTDOWN : Inport  Port=7
  ADD : Subsystem
  COILOUTF : Subsystem
  DAMP : Subsystem
  Demux9 : Demux
  FF : Subsystem
  LVDTINF : Subsystem
  MASTER : Subsystem
  Mux9 : Mux  Inputs=2
  SC : Subsystem
  Sum : Sum  Inputs=++|
  TEST : Subsystem
  WATCHDOG : cdsFunctionCall/Subsystem  Tag=cdsFunctionCall  Description=inline OSEMWATCHDOG /opt/rtcds/userapps/release/vis/common/src/WATCHDOG.c
      settings: AttributesFormatString=%<Tag>\n%<Description>
  WD : VIS_LIB/WD_GAS
  WDMON : VIS_LIB/WDMON
  GAS_CTR_OUT : Outport
  WD_STAT_OUT : Outport  Port=2
  DAMP_STAT_OUT : Outport  Port=3
  wires:
  Demux9/2 -> WDMON/2
  Demux9/3 -> WDMON/3
  WD/1 -> Mux9/2
  COILOUTF/1(Out1) -> MASTER/1(GAS_In)
  LVDTINF/1(Out1) -> Sum/2
  WATCHDOG/1 -> Demux9/1
  Demux9/4 -> WDMON/4
  Mux9/1 -> WATCHDOG/1
  DAMP/2(DAMP_STATE_Out) -> [DAMPSTATE]
  DAMP/1(F0_Out) -> ADD/3(DAMP_In)
  MASTERSW_IN/1 -> MASTER/2(MASTERSWITCH)
  [WDBLOCKFLAG] -> WD_STAT_OUT/1
  [DAMPSTATE] -> DAMP_STAT_OUT/1
  TEST/1(F0_Out) -> ADD/2(TEST_In)
  SHUTDOWN/1 -> MASTER/3(WDFLAG)
  MASTER/1(GAS_Out) -> GAS_CTR_OUT/1
  ADD/1(GAS_MAIN_Out) -> COILOUTF/1(In1)
  Demux9/1 -> [WDBLOCKFLAG], WDMON/1
  LVDT_GAS_IN/1 -> LVDTINF/1(In1), WD/1
  COILOUT_CTRL/1 -> COILOUTF/2(In2)
  COILOUTF_MASK/1 -> COILOUTF/3(In3)
  WDRESET_IN/1 -> Mux9/1
  PEM_SEIS_Z_IN/1 -> FF/1(In1), SC/1(In1)
  SC/1(Out1) -> Sum/1
  Sum/1 -> DAMP/1(GAS_In)
  FF/1(Out1) -> ADD/1(FF_In)
